simulink model "compare_windows_static"  (R2018b)
settings: Solver=ode45  StartTime=0  StopTime=24*3600  MaxStep=600  RelTol=1e-3  EnableMultiTasking=on
libraries: carnot x7, simulink_extras x2
settings Model: Creator=drhf  LastModifiedBy=drhf
settings DataIOCC: LimitDataPoints=on  SaveFormat=Array
settings OptimizationCC: DefaultParameterBehavior=Inlined  LifeSpan=inf
settings DebuggingCC: UnderspecifiedInitializationDetection=Classic  MergeDetectMultiDrivingBlocksExec=none  SolverPrmCheckMsg=warning  SFUnexpectedBacktrackingDiag=warning  SFNoUnconditionalDefaultTransitionDiag=warning  SFExecutionAtInitializationDiag=none
settings HardwareCC: ProdBitPerPointer=32  ProdBitPerSizeT=32  ProdBitPerPtrDiffT=32  ProdLargestAtomicFloat=None  ProdIntDivRoundTo=Undefined  ProdEndianess=Unspecified  ProdWordSize=32  ProdHWDeviceType=32-bit Generic
settings ModelReferenceCC: PropagateSignalLabelsOutOfModel=off
settings SFSimCC: SimUseLocalCustomCode=off
settings RTWCC: RTWUseLocalCustomCode=off
settings CodeAppCC: StateflowObjectComments=on
settings GRTTargetCC: TargetLangStandard=C89/C90 (ANSI)  GeneratePreprocessorConditionals=Disable all
settings ConfigComp: CovMetricSettings=dw  CovHtmlReporting=on  CovSaveCumulativeToWorkspaceVar=on  CovSaveSingleToWorkspaceVar=on  CovExternalEMLEnable=off

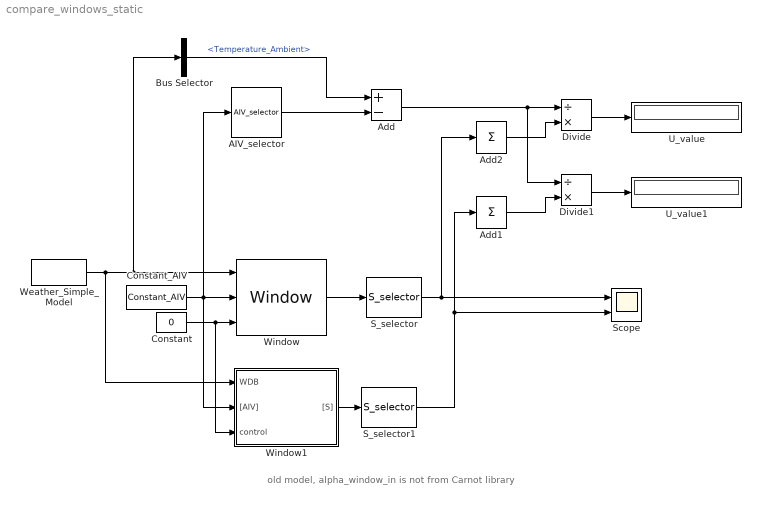
== system compare_windows_static ==
  note: old model, alpha_window_in is not from Carnot library
  AIV_selector : carnot/Outputs/AIV_selector  e1=on  e2=off  e3=off  e4=off  e5=off  e6=off  e7=off  e8=off  e9=off
      settings: SourceProductName=Carnot
  Add : Sum  Inputs=+-
  Add1 : Sum  Inputs=1
  Add2 : Sum  Inputs=1
  Bus Selector : BusSelector  OutputSignals=Temperature_Ambient
  Constant : Constant  Value=0
  Constant_AIV : carnot/Source/Ventilation/Constant_AIV  Tsens=20  Tcon=20  Trad=20  mw=0.012  mco=0.01  rhoair=1.2  cpair=1004  pair=100000  nair=0.5
      settings: SourceProductName=Carnot
  Divide : Product  Inputs=/*
  Divide1 : Product  Inputs=/*
  S_selector : carnot/Outputs/S_selector  e1=off  e2=off  e3=off  e4=off  e5=off  e6=off  e7=on  e8=on  e9=off  e10=off  e11=off  e12=off  e13=off
      settings: SourceProductName=Carnot
  S_selector1 : carnot/Outputs/S_selector  e1=off  e2=off  e3=off  e4=off  e5=off  e6=off  e7=on  e8=on  e9=off  e10=off  e11=off  e12=off  e13=off
      settings: SourceProductName=Carnot
  Scope : Scope  NumInputPorts=2
  U_value : Display
  U_value1 : Display
  Weather_Simple_Model : carnot/Weather/Weather_Simple_Model  Ibn=900  Idg=100  tamb=0  deltaTsky=0  rh=50  precip="10e-3/24/3600           % 10 mm in 24 h"  cloud=0.125  p=1013e2  vw=5.85  wdir=270  lat=60  colangle=0  colazi=0  colrot=0
      settings: SourceProductName=Carnot
  Window : carnot/Basic/Thermal_Models/Window  pos=0  windowsize=[1 1]  frame=0.1  Ug=1.8  gvalue=0.6  tauzero=0.8  numpanes=2  d=[0.004 0.004]  rho=[2500 2500]  cp="[1008  1008]"  t0=20  misc=[0.2 0.1 1 1]  shad_type=No shading  type_glazing=double glazing normal  tau_shad=0.01  bli_a=0.05  bli_b=1  bli_c=0.05  bli_d=0.05  bli_alpha=90  bli_refl=0.2
      settings: SourceProductName=Carnot
  Window1 : Subsystem  mask(window){pos=0, windowsize=[1 1], frame=0.1, Ug=1.8, gvalue=0.6, tauzero=0.8, numpanes=2, d=[0.004 0.004], rho=[2500 2500], cp=[1008  1008], t0=20, misc=[0.2 0.1 1 1], shad_type=No shading, type_glazing=Dreifach-Wärmeschutzglas, tau_shad=0.01, bli_a=0.05, bli_b=1, bli_c=0.05, bli_d=0.05, bli_alpha=90, bli_refl=0.2}
      mask prompts: pos "azimut (0=south, east = -90)"; windowsize "size of window [m] [height width]"; frame "part of frame of the surface (0..1)"; Ug "heat transfer coefficient (U-value) [W/m²K]"; gvalue "total solar energy transmittance (g-value) [0..1]"; tauzero "transmittance in visible range of the sunlight [0..1]"; numpanes "number of glass panes [1..4]"; d "thickness of glass panes [m] (vector with one element per pane)"; rho "density of glass [kg/m³] (vector with one element per pane)"; cp "capacity of glass [J/(kg*K)] (vector with one element per pane)"; t0 "initial temperature [°C]"; misc "[reflection_ground absorption_out emission_out emission_in]"; shad_type "shading type [no Shading/exterior/interior]"; type_glazing "glazing type"; tau_shad "solar transmittance of shading element [0..1]"; bli_a "a  Depth of blind blades [m]"; bli_b "b heigth of blind blades [m]"; bli_c "c distance of "b" to back end of blind blade [m]"; bli_d "d offset between blind blades [m]"; bli_alpha "blind angle  (0=closed, 90=horizontal) [0..90]"; bli_refl "optical reflectance of blind surface [0..1]"
      mask help:
      | The window model evaluates the g-value, the total energy transmission tau and the u-value to build up a two node model.
      | control input [0..1] = fraction of shading (0 - no shading,   1 - full shading)
      mask init:
      | % Geometry
      | h = windowsize(1);
      | w = windowsize(2);
      | windowsurface = h*w;
      | if length(pos) == 1
      |     pos = [90  pos 0]; % pos is [inclination azimut rotation]
      | end
      | 
      | % Optics
      | reflectground = max(0, min(1, misc(1)));
      | absorption_out = max(0, min(1, misc(2)));
      | emission_out = max(0, min(1, misc(3)));
      | emission_in = max(0, min(1, misc(4)));
      | 
      | % Thermal
      | R_norm_in = 1/8;     % h_int = 8 W/m²/K set according to ISO
      | R_norm_out = 1/25;   % h_out = 25 W/m²/K set according to ISO
      | Rwin = 1/Ug - R_norm_in - R_norm_out;
      | % C = sum(cp.*rho.*d.^2); % old equation
      | C = sum(cp.*rho.*d); % corrected equation, hf 29nov2017
      | timeconst = Rwin*C/2;
      mask Help: web(fullfile(path_carnot('help'),'WindowWithShading.html'),'-helpbrowser')
      mask TypeOptions shad_type: No shading | Exterior Screen | Interior Screen | Venetian Blind
      mask Callback shad_type:
      | switch get_param(gcb,'shad_type')
      |         case 'No shading' % nr. 1 no shading
      |             set_param(gcb,'MaskVisibilities',{'on','on','on','on','on','on','on','on','on','on','on','on','on','off','off','off','off','off','off','off','off'});
      |         case 'Exterior Screen' % nr. 2 external screen
      |             set_param(gcb,'MaskVisibilities',{'on','on','on','on','on','on','on','on','on','on','on','on','on','off','on','off','off','off','off','off','off'});
      |         case 'Interior Screen' % nr. 3 Interior Screen
      |             set_param(gcb,'MaskVisibilities',{'on','on','on','on','on','on','on','on','on','on','on','on','on','on','on','off','off','off','off','off','off'});
      |         case 'Venetian Blind' % nr. 4 venetian blind
      |             set_param(gcb,'MaskVisibilities',{'on','on','on','on','on','on','on','on','on','on','on','on','on','off','off','on','on','on','on','on','on'});
      |     end
      mask TypeOptions type_glazing: Zweifachglas normal | Zweifach-Wärmeschutzglas | Zweifach-Kombiglas 73/41 | Zweifach-Kombiglas 50/24 | Dreifachglas normal | Dreifach-Wärmeschutzglas
  wires:
  Weather_Simple_Model/1 -> Window1/1(WDB), Window/1, Bus Selector/1
  Window/1 -> S_selector/1
  S_selector/1 -> Scope/1, Add2/1
  AIV_selector/1 -> Add/2
  Add/1 -> Divide1/1, Divide/1
  Add2/1 -> Divide/2
  Divide/1 -> U_value/1
  Constant/1 -> Window1/3(control), Window/3
  Bus Selector/1 -> Add/1  "<Temperature_Ambient>"
  Constant_AIV/1 -> Window1/2("[AIV]"), Window/2, AIV_selector/1
  Divide1/1 -> U_value1/1
  Add1/1 -> Divide1/2
  S_selector1/1 -> Scope/2, Add1/1
  Window1/1("[S]") -> S_selector1/1

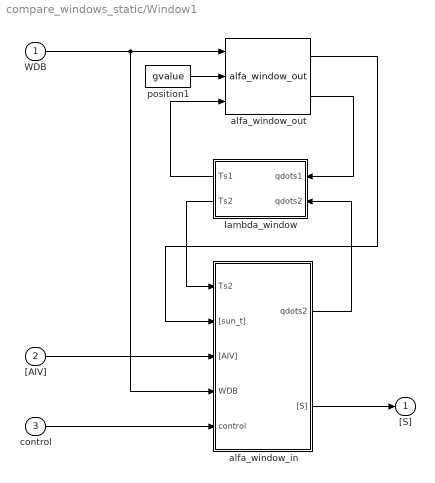
== system compare_windows_static/Window1 ==
  WDB : Inport
  "[AIV]" : Inport  Port=2
  control : Inport  Port=3
  alfa_window_in : Subsystem  mask(ALFA){}
      mask help:
      | Convective and radiative heat transfer at the INDOOR SURFACE OF A VERTICAL WINDOW with 1-4 layers (each 3 ... 8 mm thick).
      |
      | Ts  : temperature of window surface, °C,
      | [sun_t]  : sun data (incidence angle, direct and diffuse radiation
      |     at tilted window surface),
      | [AIV]  : conditions of zone node,
      | qdots  : specific heat flow into window construction, W/m^2,
      | [S]  : heat and air flow to zone node.
  alfa_window_out : carnot/Basic/Heat_Transfer/alfa_window_out  pos=pos  absorption_out=absorption_out  emission_out=emission_out  frame=frame
      settings: SourceProductName=Carnot
  lambda_window : Subsystem  mask(LAMBDA){}
      mask help:
      | Heat conduction through a transparent component (window).
      |
      | qdots1	: specific heat flow vertical on surface 1, W/m²
      | qdots2	: specific heat flow vertical on surface 2, W/m²
      | Ts1	: temperature of surface 1, °C
      | Ts2	: temperature of surface 2, °C
      |
      | NOTE CONVENTION for INPUT NUMBER:
      | "1"	  indoor surface of an outer window OR
      | 	  surface "a" of an inner window OR
      |  	  surface "f" of a glass floor
      |
      | "2"	  outdoor surface of a window OR
      | 	  surface "b" of an inner window OR
      |  	  surface "c" of a glass ceiling
  position1 : Constant  Value=gvalue
  "[S]" : Outport
  wires:
  lambda_window/1(Ts1) -> alfa_window_out/3
  WDB/1 -> alfa_window_out/1, alfa_window_in/4(WDB)
  "[AIV]"/1 -> alfa_window_in/3("[AIV]")
  alfa_window_in/1(qdots2) -> lambda_window/2(qdots2)
  alfa_window_in/2("[S]") -> "[S]"/1
  alfa_window_out/2 -> lambda_window/1(qdots1)
  alfa_window_out/1 -> alfa_window_in/2("[sun_t]")
  control/1 -> alfa_window_in/5(control)
  position1/1 -> alfa_window_out/2
  lambda_window/2(Ts2) -> alfa_window_in/1(Ts2)

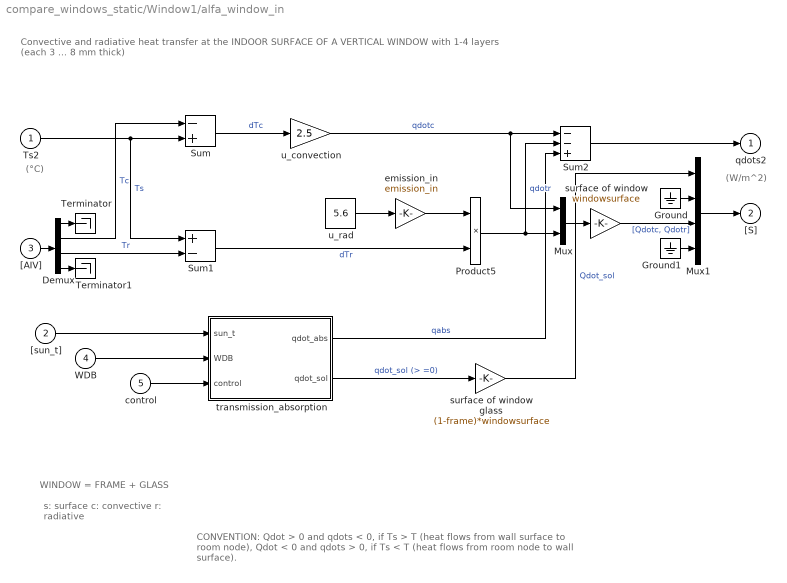
== system compare_windows_static/Window1/alfa_window_in ==
  note: (W/m^2)
  note: CONVENTION:
      | Qdot > 0 and qdots < 0, if Ts > T (heat flows from wall surface to room node),
      | Qdot < 0 and qdots > 0, if Ts < T (heat flows from room node to wall surface).
  note: s: surface
      | c: convective
      | r: radiative
  note: WINDOW = FRAME + GLASS
  note: Convective and radiative heat transfer at the INDOOR SURFACE OF A VERTICAL WINDOW
      | with 1-4 layers (each 3 ... 8 mm thick)
  note: (°C)
  Ts2 : Inport
  "[sun_t]" : Inport  Port=2
  "[AIV]" : Inport  Port=3
  WDB : Inport  Port=4
  control : Inport  Port=5
  Demux : Demux  Outputs=[1 1 1 6]
  Ground : Ground
  Ground1 : Ground
  Mux : Mux  Inputs=2
  Mux1 : Mux  Inputs=[1 5 2 5]
  Product5 : Product  SaturateOnIntegerOverflow=on  RndMeth=Zero  InputSameDT=on  OutDataTypeStr=Inherit: Same as first input
  Sum : Sum  Inputs=-+  SaturateOnIntegerOverflow=on  InputSameDT=on  OutDataTypeStr=Inherit: Same as first input
  Sum1 : Sum  Inputs=+-  SaturateOnIntegerOverflow=on  InputSameDT=on  OutDataTypeStr=Inherit: Same as first input
  Sum2 : Sum  Inputs=--+  SaturateOnIntegerOverflow=on  InputSameDT=on  OutDataTypeStr=Inherit: Same as first input
  Terminator : Terminator
  Terminator1 : Terminator
  emission_in : Gain  Gain=emission_in  SaturateOnIntegerOverflow=on  OutDataTypeStr=Inherit: Same as input  ParamDataTypeStr=Inherit: Same as input
  surface of window : Gain  Gain=windowsurface  SaturateOnIntegerOverflow=on  OutDataTypeStr=Inherit: Same as input  ParamDataTypeStr=Inherit: Same as input
  surface of window glass : Gain  Gain=(1-frame)*windowsurface  SaturateOnIntegerOverflow=on  OutDataTypeStr=Inherit: Same as input  ParamDataTypeStr=Inherit: Same as input
  transmission_absorption : Subsystem
  u_convection : Gain  Gain=2.5  SaturateOnIntegerOverflow=on  OutDataTypeStr=Inherit: Same as input  ParamDataTypeStr=Inherit: Same as input
  u_rad : Constant  Value=5.6
  qdots2 : Outport
  "[S]" : Outport  Port=2
  wires:
  Ground1/1 -> Mux1/4
  Ground/1 -> Mux1/2
  Mux1/1 -> "[S]"/1
  Sum2/1 -> qdots2/1
  Demux/4 -> Terminator1/1
  "[AIV]"/1 -> Demux/1
  Demux/1 -> Terminator/1
  Mux/1 -> surface of window/1
  emission_in/1 -> Product5/1
  Sum1/1 -> Product5/2  "dTr"
  u_rad/1 -> emission_in/1
  Ts2/1 -> Sum/2, Sum1/1  "Ts"
  Product5/1 -> Mux/2, Sum2/2  "qdotr"
  u_convection/1 -> Sum2/1, Mux/1  "qdotc"
  "[sun_t]"/1 -> transmission_absorption/1(sun_t)
  surface of window glass/1 -> Mux1/1  "Qdot_sol"
  surface of window/1 -> Mux1/3  "[Qdotc, Qdotr]"
  Demux/2 -> Sum/1  "Tc"
  Sum/1 -> u_convection/1  "dTc"
  Demux/3 -> Sum1/2  "Tr"
  transmission_absorption/2(qdot_sol) -> surface of window glass/1  "qdot_sol (> =0)"
  transmission_absorption/1(qdot_abs) -> Sum2/3  "qabs"
  WDB/1 -> transmission_absorption/2(WDB)
  control/1 -> transmission_absorption/3(control)

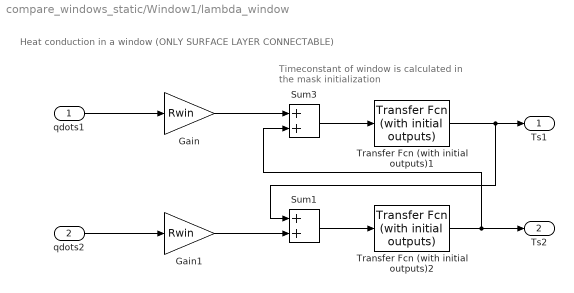
== system compare_windows_static/Window1/lambda_window ==
  note: Timeconstant of window is calculated
      | in the mask initialization
  note: Heat conduction in a window (ONLY SURFACE LAYER CONNECTABLE)
  qdots1 : Inport
  qdots2 : Inport  Port=2
  Gain : Gain  Gain=Rwin
  Gain1 : Gain  Gain=Rwin
  Sum1 : Sum  SaturateOnIntegerOverflow=on  InputSameDT=on  OutDataTypeStr=Inherit: Same as first input
  Sum3 : Sum  SaturateOnIntegerOverflow=on  InputSameDT=on  OutDataTypeStr=Inherit: Same as first input
  Transfer Fcn (with initial outputs)1 : simulink_extras/Additional Linear/Transfer Fcn (with initial outputs)  N=[1]  D=[timeconst 1]  Y0=t0  U0=t0
  Transfer Fcn (with initial outputs)2 : simulink_extras/Additional Linear/Transfer Fcn (with initial outputs)  N=[1]  D=[timeconst 1]  Y0=t0  U0=t0
  Ts1 : Outport
  Ts2 : Outport  Port=2
  wires:
  Gain1/1 -> Sum1/2
  Gain/1 -> Sum3/1
  Sum1/1 -> Transfer Fcn (with initial outputs)2/1
  qdots2/1 -> Gain1/1
  Sum3/1 -> Transfer Fcn (with initial outputs)1/1
  qdots1/1 -> Gain/1
  Transfer Fcn (with initial outputs)1/1 -> Ts1/1, Sum1/1
  Transfer Fcn (with initial outputs)2/1 -> Sum3/2, Ts2/1

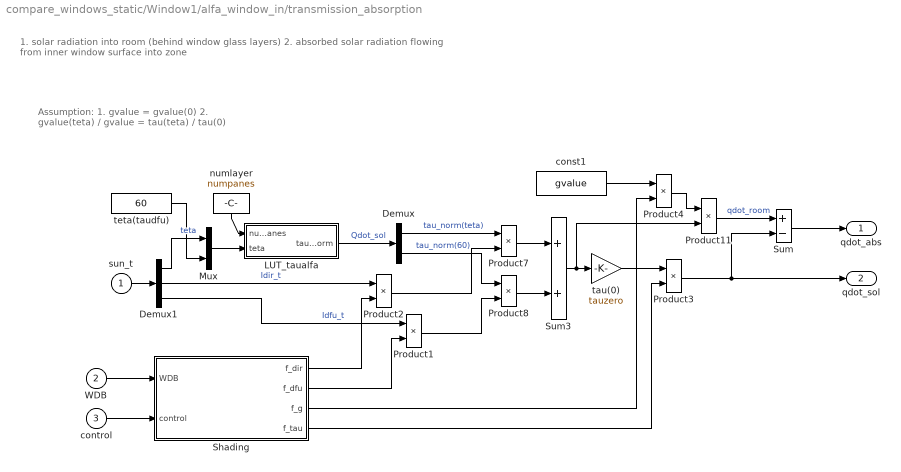
== system compare_windows_static/Window1/alfa_window_in/transmission_absorption ==
  note: 1. solar radiation into room (behind window glass layers)
      | 2. absorbed solar radiation flowing from inner window surface into zone
  note: Assumption:
      | 1. gvalue = gvalue(0)
      | 2. gvalue(teta) / gvalue = tau(teta) / tau(0)
  sun_t : Inport
  WDB : Inport  Port=2
  control : Inport  Port=3
  Demux : Demux  Outputs=2
  Demux1 : Demux  Outputs=3
  LUT_taualfa : Subsystem  mask(LOOK UP TABLE){}
      mask help:
      | Normalized RADIATION TRANSMISSION COEFFICIENT of a window glass layer stack with 1, 2, 3 or 4 layers depending on the incidence angle.
      |
      | teta		: incidence angle = angle between surface normal and
      | 	                incidence direction, degree
      | numlayer	: number of layers within the window glass, [1,4].
      | tau		: transmission of glass layer stack, [0,1]
      |
      | NOTE: This block is defined for pane thickness between 3 and 6 mm.
  Mux : Mux  Inputs=2
  Product{1..4,7..8} (6 alike) : Product  SaturateOnIntegerOverflow=on  RndMeth=Zero  InputSameDT=on  OutDataTypeStr=Inherit: Same as first input
  Product11 : Product  Inputs=**  SaturateOnIntegerOverflow=on  RndMeth=Zero  InputSameDT=on  OutDataTypeStr=Inherit: Same as first input
  Shading : Subsystem
  Sum : Sum  Inputs=+-  SaturateOnIntegerOverflow=on  InputSameDT=on  OutDataTypeStr=Inherit: Same as first input
  Sum3 : Sum  SaturateOnIntegerOverflow=on  InputSameDT=on  OutDataTypeStr=Inherit: Same as first input
  const1 : Constant  Value=gvalue
  numlayer : Constant  Value=numpanes
  tau(0) : Gain  Gain=tauzero  SaturateOnIntegerOverflow=on  OutDataTypeStr=Inherit: Same as input  ParamDataTypeStr=Inherit: Same as input
  teta(taudfu) : Constant  Value=60
  qdot_abs : Outport
  qdot_sol : Outport  Port=2
  wires:
  Mux/1 -> LUT_taualfa/2(teta)
  numlayer/1 -> LUT_taualfa/1(numlpanes)
  teta(taudfu)/1 -> Mux/2
  Demux1/1 -> Mux/1  "teta"
  Sum/1 -> qdot_abs/1
  Product11/1 -> Sum/1  "qdot_room"
  Demux/2 -> Product8/1  "tau_norm(60)"
  Sum3/1 -> tau(0)/1, Product11/2
  Product8/1 -> Sum3/2
  Product7/1 -> Sum3/1
  Demux/1 -> Product7/1  "tau_norm(teta)"
  LUT_taualfa/1(tau_norm) -> Demux/1  "Qdot_sol"
  sun_t/1 -> Demux1/1
  tau(0)/1 -> Product3/1
  Product3/1 -> Sum/2, qdot_sol/1
  Demux1/3 -> Product1/1  "Idfu_t"
  Product1/1 -> Product8/2
  Demux1/2 -> Product2/1  "Idir_t"
  Product2/1 -> Product7/2
  Shading/1(f_dir) -> Product2/2
  Shading/2(f_dfu) -> Product1/2
  Shading/4(f_tau) -> Product3/2
  Product4/1 -> Product11/1
  const1/1 -> Product4/1
  Shading/3(f_g) -> Product4/2
  WDB/1 -> Shading/1(WDB)
  control/1 -> Shading/2(control)

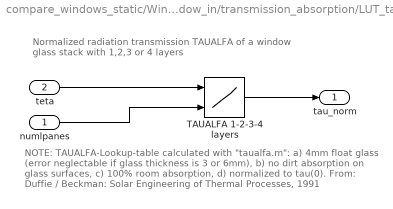
== system compare_windows_static/Window1/alfa_window_in/transmission_absorption/LUT_taualfa ==
  note: Normalized radiation transmission TAUALFA
      | of a window glass stack with 1,2,3 or 4 layers
  note: NOTE:
      | TAUALFA-Lookup-table calculated with "taualfa.m":
      |   a) 4mm float glass (error neglectable if glass thickness is 3 or 6mm),
      |   b) no dirt absorption on glass surfaces,
      |   c) 100% room absorption,
      |   d) normalized to tau(0).
      |
      | From: Duffie / Beckman: Solar Engineering of Thermal Processes, 1991
  numlpanes : Inport
  teta : Inport  Port=2
  TAUALFA 1-2-3-4 layers : Lookup2D  RowIndex=[0:10:90]  ColumnIndex=[1:4]  Table="[1  1  1  1;.99955 .99912  .9987 .99827;.99787  .9961 .99449 .99298;.99364 .98941 .98618 .98366;.98364 .97519 .97041 .96824;.9601 .94337 .93638 .93624;.90423 .86634 .84734 .84064;.77129 .67843 .61507 .56891;.47436  .3235 .22952 .16682;0  0  0  0]"  SaturateOnIntegerOverflow=on  InputSameDT=on
  tau_norm : Outport
  wires:
  TAUALFA 1-2-3-4 layers/1 -> tau_norm/1
  numlpanes/1 -> TAUALFA 1-2-3-4 layers/2
  teta/1 -> TAUALFA 1-2-3-4 layers/1

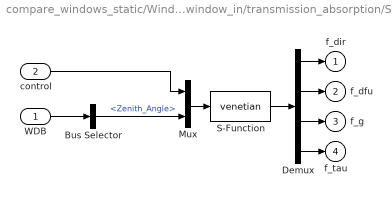
== system compare_windows_static/Window1/alfa_window_in/transmission_absorption/Shading ==
  WDB : Inport
  control : Inport  Port=2
  Bus Selector : BusSelector  OutputSignals=Zenith_Angle
  Demux : Demux
  Mux : Mux  Inputs=2
  S-Function : S-Function  FunctionName=venetian  Parameters=bli_a, bli_b, bli_c, bli_d, bli_alpha, bli_refl, shad_type, type_glazing, tau_shad  SFunctionDeploymentMode=off  EnableBusSupport=off
  f_dir : Outport
  f_dfu : Outport  Port=2
  f_g : Outport  Port=3
  f_tau : Outport  Port=4
  wires:
  Demux/4 -> f_tau/1
  Demux/3 -> f_g/1
  Demux/2 -> f_dfu/1
  Demux/1 -> f_dir/1
  S-Function/1 -> Demux/1
  Mux/1 -> S-Function/1
  control/1 -> Mux/1
  Bus Selector/1 -> Mux/2  "<Zenith_Angle>"
  WDB/1 -> Bus Selector/1
